simulink model "task3"  (R2023b)
settings: Solver=VariableStepAuto  StartTime=0.0  StopTime=10.0  RelTol=1e-3

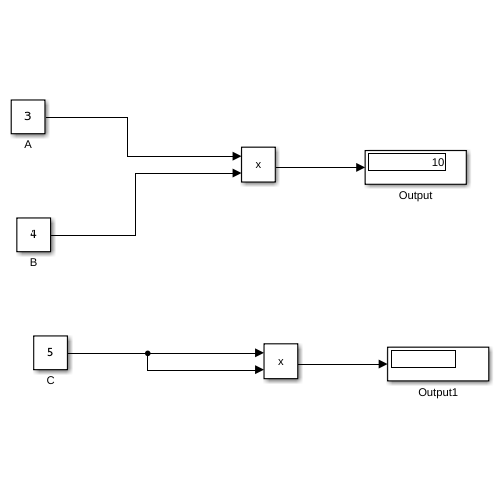
[thumbnail: Simulink's stored preview of the top-level diagram]
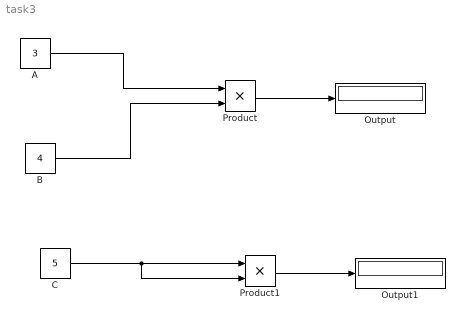
== system task3 ==
  A : Constant  Value=3
  B : Constant  Value=4
  C : Constant  Value=5
  Output : Display
  Output1 : Display
  Product : Product
  Product1 : Product
  wires:
  A/1 -> Product/1
  B/1 -> Product/2
  Product/1 -> Output/1
  C/1 -> Product1/2, Product1/1
  Product1/1 -> Output1/1
